simulink subsystem "test_attit_cntrl"  (R2022a)
settings: Solver=VariableStepAuto  StartTime=0.0  StopTime=10.0  RelTol=1e-3
libraries: aerolibutil x2
settings Model: Creator=samuel  LastModifiedBy=samuel

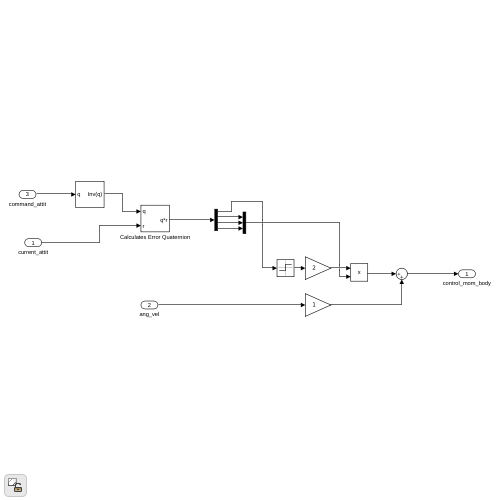
[thumbnail: Simulink's stored preview of the top-level diagram]
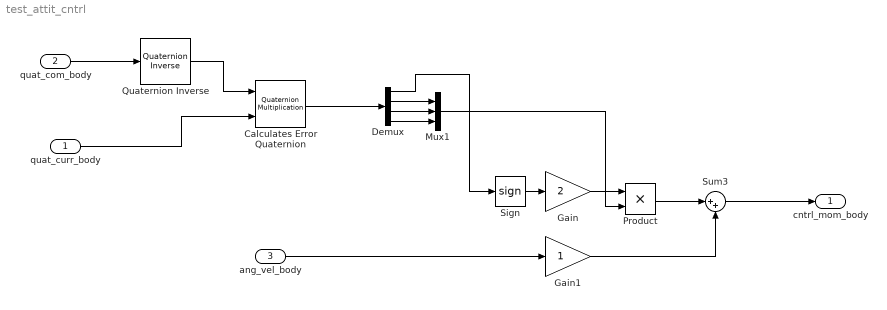
== system test_attit_cntrl ==
  quat_curr_body : Inport
  quat_com_body : Inport  Port=2
  ang_vel_body : Inport  Port=3
  Calculates Error Quaternion : aerolibutil/Quaternion Multiplication
  Demux : Demux
  Gain : Gain  Gain=2
  Gain1 : Gain
  Mux1 : Mux  Inputs=3
  Product : Product
  Quaternion Inverse : aerolibutil/Quaternion Inverse
  Sign : Signum
  Sum3 : Sum  Inputs=|++
  cntrl_mom_body : Outport
  wires:
  Sum3/1 -> cntrl_mom_body/1
  Sign/1 -> Gain/1
  quat_curr_body/1 -> Calculates Error Quaternion/2
  Demux/3 -> Mux1/2
  Gain1/1 -> Sum3/2
  Product/1 -> Sum3/1
  Demux/1 -> Sign/1
  Gain/1 -> Product/1
  ang_vel_body/1 -> Gain1/1
  quat_com_body/1 -> Quaternion Inverse/1
  Mux1/1 -> Product/2
  Demux/4 -> Mux1/3
  Quaternion Inverse/1 -> Calculates Error Quaternion/1
  Demux/2 -> Mux1/1
  Calculates Error Quaternion/1 -> Demux/1
